simulink model "session2task1"  (R2018b)
settings: Solver=FixedStepDiscrete  StartTime=0.0  StopTime=10.0  RelTol=1e-3
settings Model: Creator=ayamu  LastModifiedBy=ayamu
settings OptimizationCC: DefaultParameterBehavior=Inlined  EnhancedBackFolding=on  PassReuseOutputArgsAs=Individual arguments  OptimizeBlockOrder=speed  DifferentSizesBufferReuse=on  OptimizationCustomize=off
settings DebuggingCC: UnderspecifiedInitializationDetection=Classic  MergeDetectMultiDrivingBlocksExec=none  ParameterTunabilityLossMsg=error
settings ModelReferenceCC: PropagateSignalLabelsOutOfModel=off
settings SFSimCC: MATLABDynamicMemAlloc=off
settings RTWCC: SystemTargetFile=ert.tlc  GenCodeOnly=on  TemplateMakefile=ert_default_tmf  GenerateReport=on  IncludeHyperlinkInReport=on  LaunchReport=on  GenerateTraceInfo=on  GenerateTraceReport=on  GenerateTraceReportSl=on  GenerateTraceReportSf=on  GenerateTraceReportEml=on
settings CodeAppCC: ForceParamTrailComments=on  IgnoreCustomStorageClasses=off  OperatorAnnotations=on  SimulinkDataObjDesc=on  SFDataObjDesc=on  InsertBlockDesc=on
settings ERTTargetCC: TargetLangStandard=C99 (ISO)  GenerateSampleERTMain=on  InlinedParameterPlacement=NonHierarchical  ERTCustomFileTemplate=example_file_process.tlc

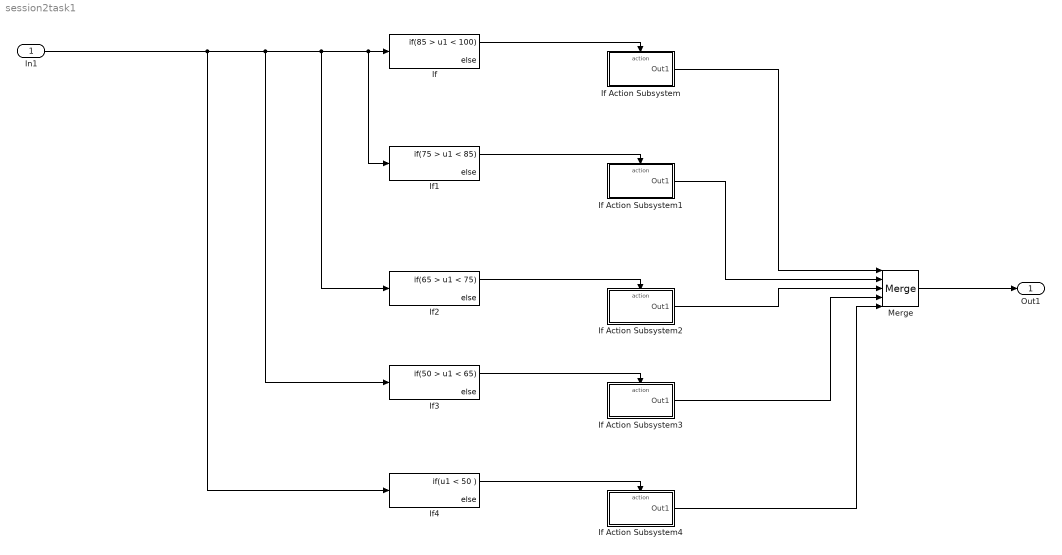
== system session2task1 ==
  In1 : Inport
  If : If  IfExpression=85 > u1 < 100
  If Action Subsystem : Subsystem  TreatAsAtomicUnit=on
  If Action Subsystem1 : Subsystem  TreatAsAtomicUnit=on
  If Action Subsystem2 : Subsystem  TreatAsAtomicUnit=on
  If Action Subsystem3 : Subsystem  TreatAsAtomicUnit=on
  If Action Subsystem4 : Subsystem  TreatAsAtomicUnit=on
  If1 : If  IfExpression=75 > u1 < 85
  If2 : If  IfExpression=65 > u1 < 75
  If3 : If  IfExpression=50 > u1 < 65
  If4 : If  IfExpression=u1 < 50
  Merge : Merge  Inputs=5
  Out1 : Outport
  wires:
  If/1 -> If Action Subsystem/Action
  If1/1 -> If Action Subsystem1/Action
  If2/1 -> If Action Subsystem2/Action
  If3/1 -> If Action Subsystem3/Action
  If4/1 -> If Action Subsystem4/Action
  Merge/1 -> Out1/1
  If Action Subsystem/1(Out1) -> Merge/1
  If Action Subsystem1/1(Out1) -> Merge/2
  If Action Subsystem2/1(Out1) -> Merge/3
  If Action Subsystem3/1(Out1) -> Merge/4
  If Action Subsystem4/1(Out1) -> Merge/5
  In1/1 -> If4/1, If1/1, If/1, If2/1, If3/1

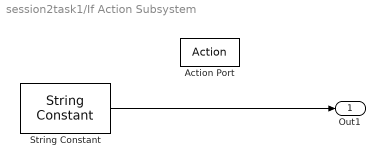
== system session2task1/If Action Subsystem ==
  Action Port : ActionPort  ActionType=then
  String Constant : StringConstant  String="\"Excellent\""
  Out1 : Outport
  wires:
  String Constant/1 -> Out1/1

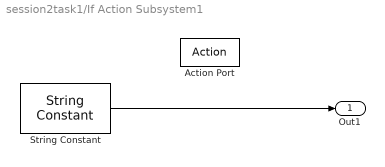
== system session2task1/If Action Subsystem1 ==
  Action Port : ActionPort  ActionType=then
  String Constant : StringConstant  String="\"VeryGood!\""
  Out1 : Outport
  wires:
  String Constant/1 -> Out1/1

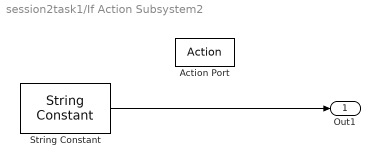
== system session2task1/If Action Subsystem2 ==
  Action Port : ActionPort  ActionType=then
  String Constant : StringConstant  String="\"Good!\""
  Out1 : Outport
  wires:
  String Constant/1 -> Out1/1

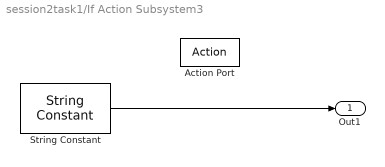
== system session2task1/If Action Subsystem3 ==
  Action Port : ActionPort  ActionType=then
  String Constant : StringConstant  String="\"Fair!\""
  Out1 : Outport
  wires:
  String Constant/1 -> Out1/1

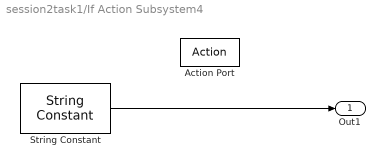
== system session2task1/If Action Subsystem4 ==
  Action Port : ActionPort  ActionType=then
  String Constant : StringConstant  String="\"Failed!\""
  Out1 : Outport
  wires:
  String Constant/1 -> Out1/1
